simulink model "Simulink_PHEV"  (R2024b)
settings: Solver=VariableStepDiscrete  StartTime=0.0  StopTime=1220  RelTol=1e-3  EnableMultiTasking=on
values from neighbouring files (symbols this model uses):
  eta_EM_map = [0.5831 0.6831 0.781 0.826 0 0 0 0 0 0.6107 0.7107 0.8049 ... (270 elements, 9x30)]    [Initial_Data.mat]
  h = []    [Initial_Data.mat]
  H_u = 42936779.9114    [Initial_Data.mat]
  P_MGB_FTP75 = [0 0 0 0 0 0 0 0 0 0 0 0 ... (1878 elements, 1878x1)]    [Initial_Data.mat]
  PMGB_NEDC = [0 0 0 0 0 0 0 0 0 0 0 0 ... (1221 elements, 1221x1)]    [Initial_Data.mat]
  rho_f = 0.843    [Initial_Data.mat]
  T_CE_max = [118.899401682 131.236739827 143.574077972 164.791588079 186.009098185 184.856709457 183.704320729 184.924497029 186.144673329 186.619186335 187.093699341 186.822549052 ... (31 elements, 1x31)]    [Initial_Data.mat]
  T_EM_max = [60 60 60 44.5714285714 32.5714285714 24 16.2857142857 11.1428571429 7.71428571429]    [Initial_Data.mat]
  V_CE_map = [0.000142 0.000157 0.000171 0.000186 0.000201 0.000215 0.000229 0.000255 0.00028 0.000299 0.000317 0.000346 ... (868 elements, 31x28)]    [Initial_Data.mat]
  w_CE_max = [125.663706144 136.135681656 146.607657168 157.079632679 167.551608191 178.023583703 188.495559215 198.967534727 209.439510239 219.911485751 230.383461263 240.855436775 ... (31 elements, 1x31)]    [Initial_Data.mat]
  w_EM_row = [0 100 200 300 400 500 600 700 800]    [Initial_Data.mat]
undefined symbols (not defined in the file or in its folder): c_BT_E1, c_BT_E2, c_BT_E3, c_BT_E4, c_BT_L1, c_BT_L2, c_BT_L3, c_BT_L4, I_BT_max, Q_BT_0, Q_BT_IC
libraries: qss_tb_library x6, mpclib x1, dspindex x1
settings Model: Creator=d_goerges  LastModifiedBy=mohammed omrez khan
settings SolverCC: AlgebraicLoopSolver=TrustRegion
settings DataIOCC: LimitDataPoints=on  SaveFormat=Array  SignalLoggingSaveFormat=ModelDataLogs  ReturnWorkspaceOutputs=off
settings OptimizationCC: ExpressionDepthLimit=2147483647  LifeSpan=inf
settings DebuggingCC: MergeDetectMultiDrivingBlocksExec=none  SolverPrmCheckMsg=warning  FcnCallInpInsideContextMsg=warning  UnconnectedInputMsg=warning  UnconnectedOutputMsg=warning  UnconnectedLineMsg=warning  StateNameClashWarn=warning  SFUnexpectedBacktrackingDiag=warning  SFNoUnconditionalDefaultTransitionDiag=warning  SFExecutionAtInitializationDiag=none  UnderSpecifiedDimensionMsg=warning  ArithmeticOperatorsInVariantConditions=warning
settings HardwareCC: ProdBitPerPointer=32  ProdBitPerSizeT=32  ProdBitPerPtrDiffT=32  ProdLargestAtomicFloat=None  ProdIntDivRoundTo=Undefined  ProdEndianess=Unspecified  ProdWordSize=32  ProdHWDeviceType=32-bit Generic
settings ModelReferenceCC: PropagateSignalLabelsOutOfModel=off
settings SFSimCC: SimUseLocalCustomCode=off  CustomCodeUndefinedFunction=UseInterfaceOnly
settings RTWCC: RTWUseLocalCustomCode=off  GPUComputeCapability=3.5
settings CodeAppCC: StateflowObjectComments=on
settings GRTTargetCC: TargetLangStandard=C89/C90 (ANSI)  CombineOutputUpdateFcns=off  GRTInterface=on
settings ConfigComp: CovMetricSettings=dw  CovSaveCumulativeToWorkspaceVar=on  CovSaveSingleToWorkspaceVar=on  CovExternalEMLEnable=off

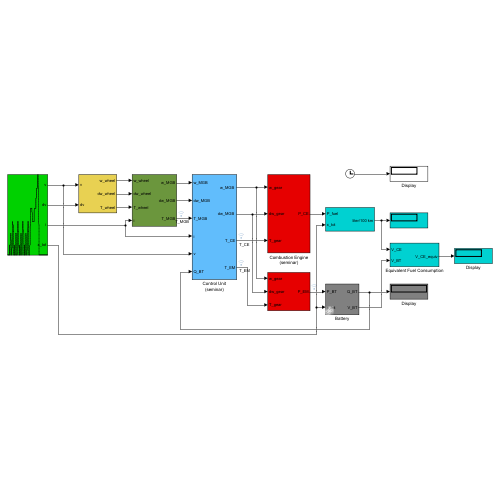
[thumbnail: Simulink's stored preview of the top-level diagram]
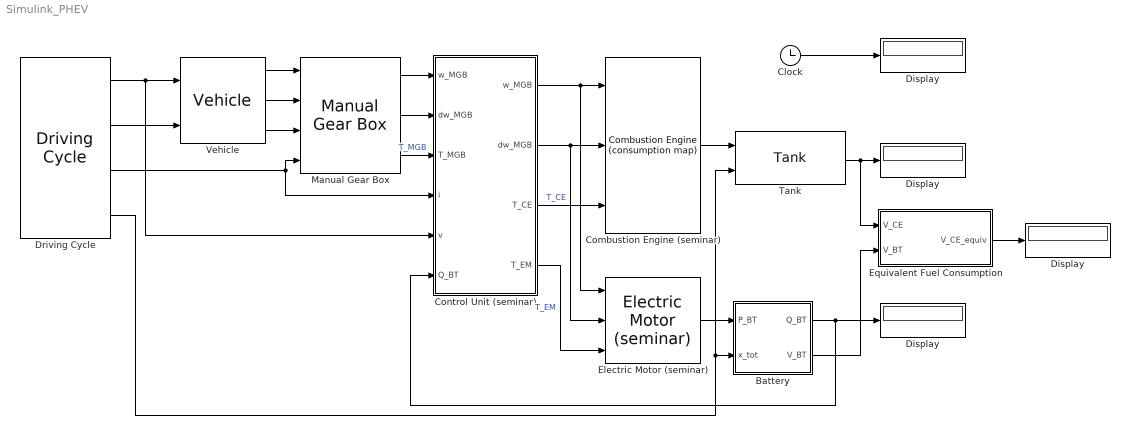
== system Simulink_PHEV ==
  "   Display   " : Display
  "  Display  " : Display
  " Display " : Display
  Battery : Subsystem  Tag=battery  AncestorBlock=qss_tb_library/Energy Buffer/Battery  mask(Battery){I_0=10, Q_BT_IC_rel=50, t_ch=2}
      mask prompts: I_0 "Energy capacity of battery [Ah]"; Q_BT_IC_rel "Initial charge of battery [%]"; t_ch "Current limit: minimum time to charge/discharge the battery [min]"
      mask help:
      | This block simulates a battery.
      | The resistance depends on the charge state and the charge/discharge current of the battery. The battery has an open circuit voltage of 130 V (fully charged).
      |
      | Input:
      | =====
      | 	x_tot	Total distance [m]
      | 	P_BT	Power from/to the battery [W]
      | 		P_BT < 0: battery charging
      | 		P_BT > 0: battery discharging
      |
      | Output:
      | ======
      | 	Q_BT	Current charge of the battery [C]
      | 	V_BT	Energy consumption [kWh/100 km]
      mask init:
      | init_BT;
  Clock : Clock
  Combustion Engine (seminar) : qss_tb_library/Energy Converter/Combustion Engine (consumption map)  Tag=combustion engine  theta_CE=0.2  w_CE_idle=105  P_CE_idle=8000  P_aux=0  ENABLE_FUEL_CUTOFF=on  T_CE_cutoff=5  P_CE_cutoff=0
  Control Unit (seminar) : Subsystem  Tag=control unit  mask(Control Unit){}
      mask help:
      | This block gives the user the opportunity to design his/her own control unit.
      |
      | The user can define the inputs and outputs  by himself/herself.
      mask init:
      | %init_control_unit;
  Display : Display
  Driving Cycle : qss_tb_library/Driving Cycle/Driving Cycle  Tag=cycle  cyclenr=Europe: NEDC  stepsize=1  autostop=on
  Electric Motor (seminar) : qss_tb_library/Energy Converter/Electric Motor (seminar)  theta_EM=0.1  P_aux=0
  Equivalent Fuel Consumption : Subsystem  mask(Equivalent Fuel Consumption){eta_BT=0.9, eta_EM=0.8, eta_CE=0.25}
      mask prompts: eta_BT "Battery efficiency [-]"; eta_EM "Motor efficiency [-]"; eta_CE "Engine efficiency [-]"
      mask help:
      | This block computes the equivalent fuel consumption.
      |
      | Input:
      | =====
      | 	V_CE    Fuel consumption [l/100 km]
      | 	V_BT    Energy consumption [kWh/100 km]
      |
      | Output:
      | ======
      | 	V_CE_equiv	Equivalent fuel consumption [l/100 km]
      mask init:
      | init_equivalent_fuel_consumption;
  Manual Gear Box : qss_tb_library/Gear System/Manual Gear Box  Tag=transmission  i_1=3.27  i_2=1.92  i_3=1.26  i_4=0.88  i_5=0.7  i_diff=3.29  e_GT=0.98  P_GT0=100  w_wheel_min=1
  Tank : qss_tb_library/Energy Source/Tank  Tag=tank  fuel=Diesel  flag_cold_start=on
  Vehicle : qss_tb_library/Vehicle/Vehicle  Tag=vehicle  m_f=1115  mt2m_f=5  A_f=2.3  d_wheel=0.576  cw=0.31  mu=0.013
  wires:
  Tank/1 -> Display/1, Equivalent Fuel Consumption/1(V_CE)
  Driving Cycle/2 -> Vehicle/2
  Driving Cycle/1 -> Vehicle/1, Control Unit (seminar)/5(v)
  Vehicle/1 -> Manual Gear Box/1
  Vehicle/2 -> Manual Gear Box/2
  Vehicle/3 -> Manual Gear Box/3
  Manual Gear Box/1 -> Control Unit (seminar)/1(w_MGB)
  Manual Gear Box/2 -> Control Unit (seminar)/2(dw_MGB)
  Manual Gear Box/3 -> Control Unit (seminar)/3(T_MGB)  "T_MGB"
  Control Unit (seminar)/1(" w_MGB ") -> Combustion Engine (seminar)/1, Electric Motor (seminar)/1
  Control Unit (seminar)/2(" dw_MGB ") -> Combustion Engine (seminar)/2, Electric Motor (seminar)/2
  Control Unit (seminar)/3(T_CE) -> Combustion Engine (seminar)/3  "T_CE"
  Control Unit (seminar)/4(T_EM) -> Electric Motor (seminar)/3  "T_EM"
  Combustion Engine (seminar)/1 -> Tank/1
  Electric Motor (seminar)/1 -> Battery/1(P_BT)
  Driving Cycle/4 -> Battery/2(x_tot), Tank/2
  Battery/1(Q_BT) -> "  Display  "/1, Control Unit (seminar)/6(Q_BT)
  Driving Cycle/3 -> Manual Gear Box/4, Control Unit (seminar)/4(i)
  Battery/2(V_BT) -> Equivalent Fuel Consumption/2(V_BT)
  Clock/1 -> " Display "/1
  Equivalent Fuel Consumption/1(V_CE_equiv) -> "   Display   "/1

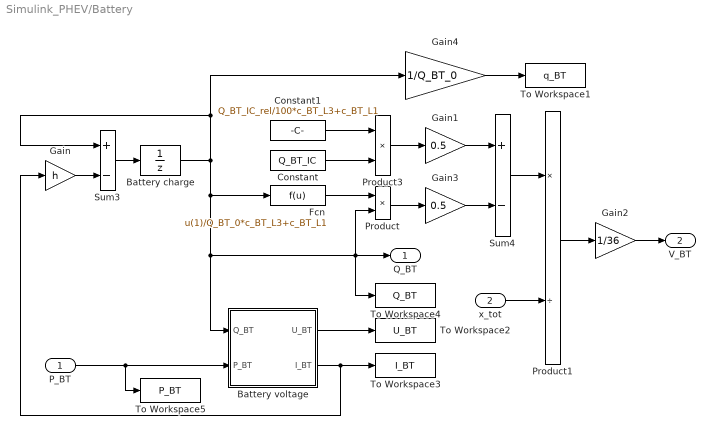
== system Simulink_PHEV/Battery ==
  P_BT : Inport
  x_tot : Inport  Port=2
  Battery charge : UnitDelay  InitialCondition=Q_BT_IC  SampleTime=h  HasFrameUpgradeWarning=on
  Battery voltage : Subsystem
  Constant : Constant  Value=Q_BT_IC
  Constant1 : Constant  Value=Q_BT_IC_rel/100*c_BT_L3+c_BT_L1
  Fcn : Fcn  Expr=u(1)/Q_BT_0*c_BT_L3+c_BT_L1
  Gain : Gain  Gain=h  SaturateOnIntegerOverflow=on  OutDataTypeStr=Inherit: Same as input  ParamDataTypeStr=Inherit: Same as input
  Gain1 : Gain  Gain=0.5  SaturateOnIntegerOverflow=on  OutDataTypeStr=Inherit: Same as input  ParamDataTypeStr=Inherit: Same as input
  Gain2 : Gain  Gain=1/36  SaturateOnIntegerOverflow=on  OutDataTypeStr=Inherit: Same as input  ParamDataTypeStr=Inherit: Same as input
  Gain3 : Gain  Gain=0.5  SaturateOnIntegerOverflow=on  OutDataTypeStr=Inherit: Same as input  ParamDataTypeStr=Inherit: Same as input
  Gain4 : Gain  Gain=1/Q_BT_0  SaturateOnIntegerOverflow=on  OutDataTypeStr=Inherit: Same as input  ParamDataTypeStr=Inherit: Same as input
  Product : Product  RndMeth=Zero
  Product1 : Product  Inputs=*/  InputSameDT=on  RndMeth=Zero  SaturateOnIntegerOverflow=on  OutDataTypeStr=Inherit: Same as first input
  Product3 : Product  RndMeth=Zero
  Sum3 : Sum  Inputs=+-  InputSameDT=on  SaturateOnIntegerOverflow=on  OutDataTypeStr=Inherit: Same as first input
  Sum4 : Sum  Inputs=+-  InputSameDT=on  SaturateOnIntegerOverflow=on  OutDataTypeStr=Inherit: Same as first input
  To Workspace1 : ToWorkspace  VariableName=q_BT  SampleTime=-1
  To Workspace2 : ToWorkspace  VariableName=U_BT  SampleTime=-1
  To Workspace3 : ToWorkspace  VariableName=I_BT  SampleTime=-1
  To Workspace4 : ToWorkspace  VariableName=Q_BT  SampleTime=-1
  To Workspace5 : ToWorkspace  VariableName=P_BT  SampleTime=-1
  Q_BT : Outport  InitialOutput=0
  V_BT : Outport  Port=2  InitialOutput=0
  wires:
  Fcn/1 -> Product/1
  Constant1/1 -> Product3/1
  Constant/1 -> Product3/2
  Gain2/1 -> V_BT/1
  Sum4/1 -> Product1/1
  Gain3/1 -> Sum4/2
  Gain1/1 -> Sum4/1
  Product/1 -> Gain3/1
  Product3/1 -> Gain1/1
  P_BT/1 -> To Workspace5/1, Battery voltage/2(P_BT)
  Gain4/1 -> To Workspace1/1
  Product1/1 -> Gain2/1
  x_tot/1 -> Product1/2
  Battery voltage/1(U_BT) -> To Workspace2/1
  Battery charge/1 -> Fcn/1, To Workspace4/1, Q_BT/1, Product/2, Battery voltage/1(Q_BT), Gain4/1, Sum3/1
  Gain/1 -> Sum3/2
  Sum3/1 -> Battery charge/1
  Battery voltage/2(I_BT) -> To Workspace3/1, Gain/1

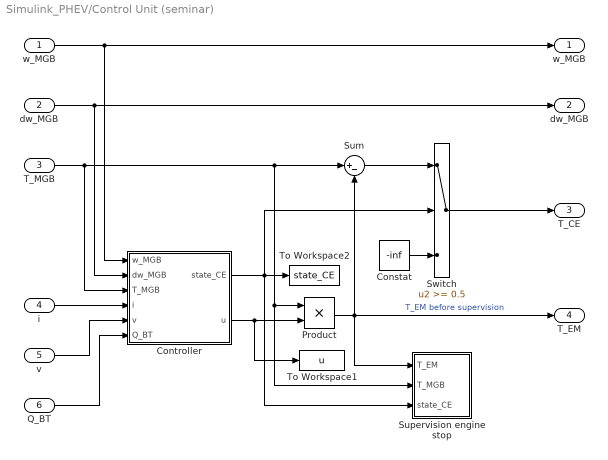
== system Simulink_PHEV/Control Unit (seminar) ==
  w_MGB : Inport
  dw_MGB : Inport  Port=2
  T_MGB : Inport  Port=3
  i : Inport  Port=4
  v : Inport  Port=5
  Q_BT : Inport  Port=6
  Constat : Constant  Value=-inf
  Controller : Subsystem  TreatAsAtomicUnit=on
  Product : Product  RndMeth=Zero
  Sum : Sum  Inputs=|+-
  Supervision engine stop : Subsystem
  Switch : Switch  Threshold=0.5  SaturateOnIntegerOverflow=off  InputSameDT=off
  To Workspace1 : ToWorkspace  VariableName=u  SampleTime=-1
  To Workspace2 : ToWorkspace  VariableName=state_CE  SampleTime=-1
  " w_MGB " : Outport  InitialOutput=0
  " dw_MGB " : Outport  Port=2  InitialOutput=0
  T_CE : Outport  Port=3  InitialOutput=0
  T_EM : Outport  Port=4  InitialOutput=0
  wires:
  dw_MGB/1 -> Controller/2(dw_MGB), " dw_MGB "/1
  w_MGB/1 -> Controller/1(w_MGB), " w_MGB "/1
  T_MGB/1 -> Controller/3(T_MGB), Sum/1, Product/1, Supervision engine stop/2(T_MGB)
  Product/1 -> Sum/2, T_EM/1, Supervision engine stop/1(T_EM)  "T_EM before supervision"
  i/1 -> Controller/4(i)
  Controller/1(state_CE) -> Switch/2, To Workspace2/1, Supervision engine stop/3(state_CE)
  Sum/1 -> Switch/1
  Switch/1 -> T_CE/1
  Constat/1 -> Switch/3
  v/1 -> Controller/5(v)
  Q_BT/1 -> Controller/6(Q_BT)
  Controller/2(u) -> To Workspace1/1, Product/2

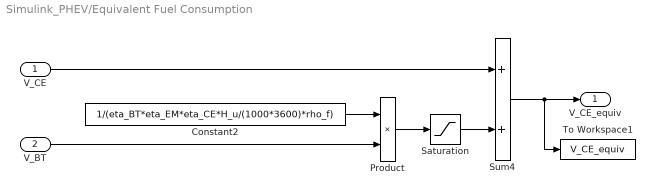
== system Simulink_PHEV/Equivalent Fuel Consumption ==
  V_CE : Inport
  V_BT : Inport  Port=2
  Constant2 : Constant  Value=1/(eta_BT*eta_EM*eta_CE*H_u/(1000*3600)*rho_f)
  Product : Product  RndMeth=Zero
  Saturation : Saturate  UpperLimit=inf  LowerLimit=0
  Sum4 : Sum  InputSameDT=on  SaturateOnIntegerOverflow=on  OutDataTypeStr=Inherit: Same as first input
  To Workspace1 : ToWorkspace  VariableName=V_CE_equiv  SampleTime=-1
  V_CE_equiv : Outport
  wires:
  Product/1 -> Saturation/1
  V_BT/1 -> Product/2
  Constant2/1 -> Product/1
  Sum4/1 -> To Workspace1/1, V_CE_equiv/1
  V_CE/1 -> Sum4/1
  Saturation/1 -> Sum4/2

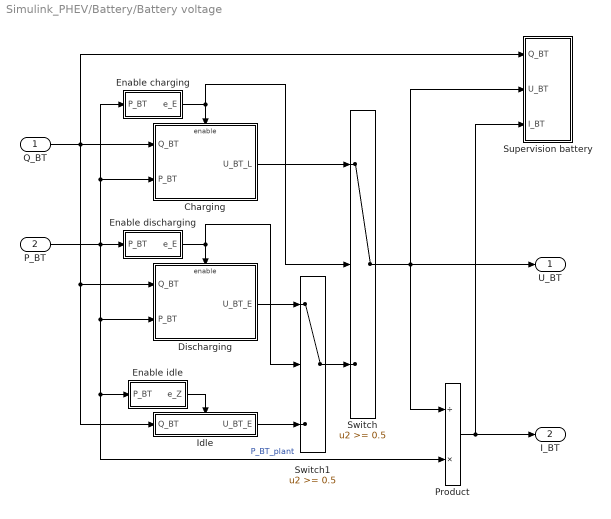
== system Simulink_PHEV/Battery/Battery voltage ==
  Q_BT : Inport
  P_BT : Inport  Port=2
  Charging : Subsystem
  Discharging : Subsystem
  Enable charging : Subsystem
  Enable discharging : Subsystem
  Enable idle : Subsystem
  Idle : Subsystem
  Product : Product  Inputs=/*  InputSameDT=on  RndMeth=Zero  SaturateOnIntegerOverflow=on  OutDataTypeStr=Inherit: Same as first input
  Supervision battery : Subsystem
  Switch : Switch  Threshold=0.5
  Switch1 : Switch  Threshold=0.5
  U_BT : Outport  InitialOutput=0
  I_BT : Outport  Port=2  InitialOutput=0
  wires:
  Switch/1 -> U_BT/1, Supervision battery/2(U_BT), Product/1
  Enable charging/1(e_E) -> Switch/2, Charging/Enable
  Q_BT/1 -> Idle/1(Q_BT), Discharging/1(Q_BT), Charging/1(Q_BT), Supervision battery/1(Q_BT)
  Product/1 -> I_BT/1, Supervision battery/3(I_BT)
  Enable discharging/1(e_E) -> Switch1/2, Discharging/Enable
  P_BT/1 -> Enable discharging/1(P_BT), Discharging/2(P_BT), Product/2, Enable idle/1(P_BT), Enable charging/1(P_BT), Charging/2(P_BT)  "P_BT_plant"
  Discharging/1(U_BT_E) -> Switch1/1
  Idle/1(U_BT_E) -> Switch1/3
  Switch1/1 -> Switch/3
  Charging/1(U_BT_L) -> Switch/1
  Enable idle/1(e_Z) -> Idle/Enable

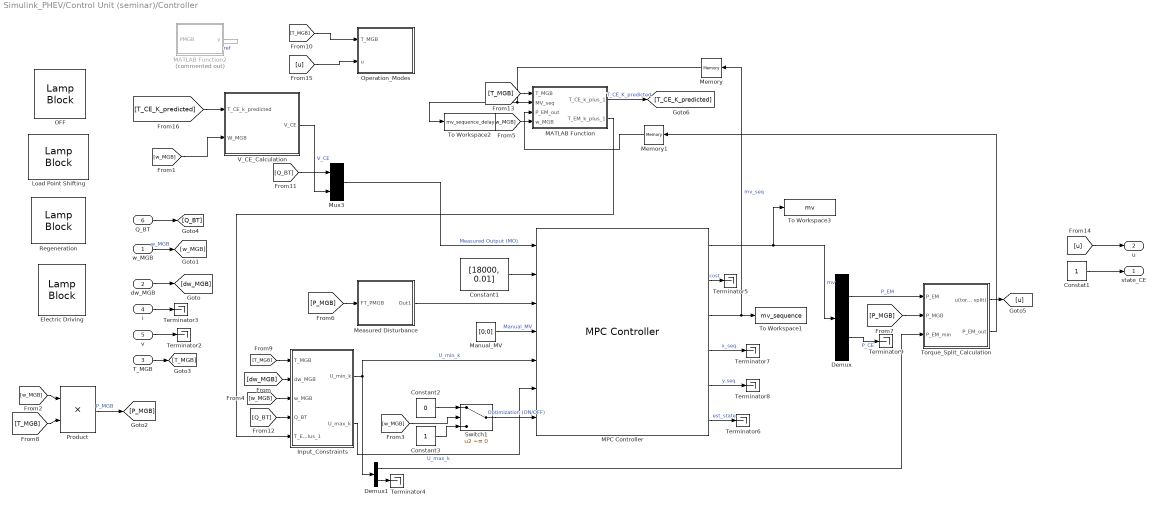
== system Simulink_PHEV/Control Unit (seminar)/Controller ==
  w_MGB : Inport
  dw_MGB : Inport  Port=2
  T_MGB : Inport  Port=3
  i : Inport  Port=4
  v : Inport  Port=5
  Q_BT : Inport  Port=6
  Constant1 : Constant  Value=[18000, 0.01]  VectorParams1D=off
  Constant2 : Constant  Value=0
  Constant3 : Constant
  Constat1 : Constant
  Demux : Demux  Outputs=2
  Demux1 : Demux  Outputs=2
  Electric Driving : LampBlock  LabelPosition=Hide
  Input_Constraints : Subsystem
  "Load Point Shifting " : LampBlock  LabelPosition=Hide
  MATLAB Function : MATLAB Function  TreatAsAtomicUnit=on
  MATLAB Function2 : MATLAB Function  Commented=on  TreatAsAtomicUnit=on
  MPC Controller : mpclib/MPC Controller  SCDEnableBlockLinearizationSpecification=on  mpcobj=mpc_object  is_multiple=0  enable_value=0  return_u0=off  updateMPCinCallerWorkspace=on  md_inport=on  mv_inport=on  uref_inport=off  return_cost=on  return_mvseq=on  return_qpstatus=off  return_xseq=on  return_state=on  return_ovseq=on  state_inport=off  umin_inport=on  umax_inport=on  ymin_inport=off  ymax_inport=off  cc_inport=off  ywt_inport=off  uwt_inport=off  duwt_inport=off  rhoeps_inport=off  pm_inport=off  MaximumP=10  HorizonChoice=FixedHorizon  n_ts=1  n_p=11  n_mv=2  n_md=1  n_ud=0  n_mo=2  n_uo=0  BlockDataType=double  SampleTimeInherited=off  switch_inport=on
  Manual_MV : Constant  Value=[0;0]  VectorParams1D=off
  Measured Disturbance : Subsystem
  Memory : Memory
  Memory1 : Memory
  Mux3 : Mux  Inputs=2
  OFF : LampBlock  LabelPosition=Hide
  Operation_Modes : Stateflow chart  TreatAsAtomicUnit=on
  Product : Product  OutDataTypeStr=double
  Regeneration : LampBlock  LabelPosition=Hide
  Switch1 : Switch  Criteria=u2 ~= 0  SaturateOnIntegerOverflow=off  InputSameDT=off
  Terminator{2..9} (8 alike) : Terminator
  To Workspace1 : ToWorkspace  VariableName=mv_sequence  SaveFormat=Timeseries  SampleTime=-1
  To Workspace2 : ToWorkspace  VariableName=mv_sequence_delay  SaveFormat=Timeseries  SampleTime=-1
  To Workspace3 : ToWorkspace  VariableName=mv  SaveFormat=Timeseries  SampleTime=-1
  Torque_Split_Calculation : Subsystem
  V_CE_Calculation : Subsystem
  state_CE : Outport  InitialOutput=0
  u : Outport  Port=2  InitialOutput=0
  wires:
  dw_MGB/1 -> [dw_MGB]
  i/1 -> Terminator3/1
  Product/1 -> [P_MGB]  "P_MGB"
  V_CE_Calculation/1(V_CE) -> Mux3/2  "V_CE"
  Input_Constraints/1(U_min_k) -> MPC Controller/5, Demux1/1  "U_min_k"
  Input_Constraints/2(U_max_k) -> MPC Controller/6  "U_max_k"
  Demux/1 -> Torque_Split_Calculation/1(P_EM)  "P_EM"
  Mux3/1 -> MPC Controller/1  "Measured Output (MO)"
  Constant1/1 -> MPC Controller/2
  v/1 -> Terminator2/1
  MPC Controller/1 -> To Workspace3/1, Demux/1  "mv"
  Manual_MV/1 -> MPC Controller/4  "Manual_MV"
  Demux/2 -> Terminator9/1  "P_CE"
  Switch1/1 -> MPC Controller/7  "Optimization (ON/OFF)"
  Constant2/1 -> Switch1/1
  Constant3/1 -> Switch1/3
  Demux1/1 -> Torque_Split_Calculation/3(P_EM_min)
  Demux1/2 -> Terminator4/1
  MPC Controller/5 -> Terminator8/1  "y.seq"
  MPC Controller/3 -> Memory/1, To Workspace1/1  "mv_seq"
  MPC Controller/6 -> Terminator6/1  "est_state"
  MPC Controller/4 -> Terminator7/1  "x_seq"
  MPC Controller/2 -> Terminator5/1  "cost"
  Memory/1 -> To Workspace2/1, MATLAB Function/2(MV_seq)
  Constat1/1 -> state_CE/1
  MATLAB Function/2(T_EM_k_plus_1) -> Input_Constraints/5(T_EM_k_plus_1)
  MATLAB Function2/1(y) -> ?  "ref"
  [dw_MGB] -> Input_Constraints/2(dw_MGB)
  w_MGB/1 -> [w_MGB]  "w_MGB"
  [w_MGB] -> V_CE_Calculation/2(W_MGB)
  [w_MGB] -> Product/1
  [w_MGB] -> Switch1/2
  [w_MGB] -> Input_Constraints/3(w_MGB)
  [w_MGB] -> MATLAB Function/4(w_MGB)
  [P_MGB] -> Measured Disturbance/1(FT_PMGB)
  [P_MGB] -> Torque_Split_Calculation/2(P_MGB)
  T_MGB/1 -> [T_MGB]
  [T_MGB] -> Product/2
  [T_MGB] -> Input_Constraints/1(T_MGB)
  [T_MGB] -> Operation_Modes/1(T_MGB)
  Measured Disturbance/1(Out1) -> MPC Controller/3
  Q_BT/1 -> [Q_BT]
  [Q_BT] -> Mux3/1
  [Q_BT] -> Input_Constraints/4(Q_BT)
  Memory1/1 -> MATLAB Function/3(P_EM_out)
  [T_MGB] -> MATLAB Function/1(T_MGB)
  Torque_Split_Calculation/2(P_EM_out) -> Memory1/1
  Torque_Split_Calculation/1(u(torque split)) -> [u]
  [u] -> u/1
  [u] -> Operation_Modes/2(u)
  MATLAB Function/1(T_CE_k_plus_1) -> [T_CE_K_predicted]  "T_CE_K_predicted"
  [T_CE_K_predicted] -> V_CE_Calculation/1(T_CE_k_predicted)

== system Simulink_PHEV/Control Unit (seminar)/Supervision engine stop ==
  T_EM : Inport
  T_MGB : Inport  Port=2
  state_CE : Inport  Port=3
  Interpreted MATLAB Function : MATLABFcn  MATLABFcn=supervision_engine_stop
  Mux : Mux  Inputs=3
  Stop Simulation : Stop
  wires:
  T_MGB/1 -> Mux/2
  T_EM/1 -> Mux/1
  state_CE/1 -> Mux/3
  Mux/1 -> Interpreted MATLAB Function/1
  Interpreted MATLAB Function/1 -> Stop Simulation/1  "Overload_supervision"

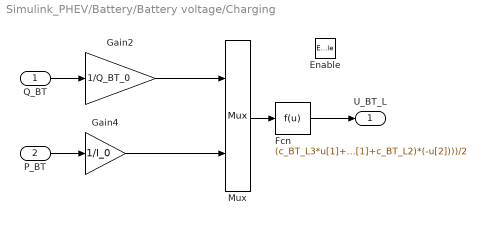
== system Simulink_PHEV/Battery/Battery voltage/Charging ==
  Q_BT : Inport
  P_BT : Inport  Port=2
  Enable : EnablePort
  Fcn : Fcn  Expr=(c_BT_L3*u[1]+c_BT_L1+sqrt((c_BT_L3*u[1]+c_BT_L1)^2+4*(c_BT_L4*u[1]+c_BT_L2)*(-u[2])))/2
  Gain2 : Gain  Gain=1/Q_BT_0  SaturateOnIntegerOverflow=on  OutDataTypeStr=Inherit: Same as input  ParamDataTypeStr=Inherit: Same as input
  Gain4 : Gain  Gain=1/I_0  SaturateOnIntegerOverflow=on  OutDataTypeStr=Inherit: Same as input  ParamDataTypeStr=Inherit: Same as input
  Mux : Mux  Inputs=2
  U_BT_L : Outport  InitialOutput=0
  wires:
  Fcn/1 -> U_BT_L/1
  Mux/1 -> Fcn/1
  P_BT/1 -> Gain4/1
  Q_BT/1 -> Gain2/1
  Gain2/1 -> Mux/1
  Gain4/1 -> Mux/2

== system Simulink_PHEV/Battery/Battery voltage/Discharging ==
  note: P/I_0
  note: q
  Q_BT : Inport
  P_BT : Inport  Port=2
  Enable : EnablePort
  Fcn : Fcn  Expr=(c_BT_E3*u[1]+c_BT_E1+sqrt((c_BT_E3*u[1]+c_BT_E1)^2+4*(c_BT_E4*u[1]+c_BT_E2)*(-u[2])))/2
  Gain4 : Gain  Gain=1/Q_BT_0  SaturateOnIntegerOverflow=on  OutDataTypeStr=Inherit: Same as input  ParamDataTypeStr=Inherit: Same as input
  Gain5 : Gain  Gain=1/I_0  SaturateOnIntegerOverflow=on  OutDataTypeStr=Inherit: Same as input  ParamDataTypeStr=Inherit: Same as input
  Mux : Mux  Inputs=2
  U_BT_E : Outport  InitialOutput=0
  wires:
  Mux/1 -> Fcn/1
  Gain5/1 -> Mux/2
  Gain4/1 -> Mux/1
  P_BT/1 -> Gain5/1
  Q_BT/1 -> Gain4/1
  Fcn/1 -> U_BT_E/1

== system Simulink_PHEV/Battery/Battery voltage/Enable charging ==
  P_BT : Inport
  Gain : Gain  Gain=-1  SaturateOnIntegerOverflow=on  OutDataTypeStr=Inherit: Same as input  ParamDataTypeStr=Inherit: Same as input
  Saturation : Saturate  UpperLimit=0  LowerLimit=-inf
  Sign : Signum
  e_E : Outport  InitialOutput=0
  wires:
  Gain/1 -> Sign/1
  Saturation/1 -> Gain/1
  Sign/1 -> e_E/1
  P_BT/1 -> Saturation/1

== system Simulink_PHEV/Battery/Battery voltage/Enable discharging ==
  P_BT : Inport
  Saturation : Saturate  UpperLimit=inf  LowerLimit=0
  Sign : Signum
  e_E : Outport  InitialOutput=0
  wires:
  Saturation/1 -> Sign/1
  Sign/1 -> e_E/1
  P_BT/1 -> Saturation/1

== system Simulink_PHEV/Battery/Battery voltage/Enable idle ==
  P_BT : Inport
  Abs : Abs
  Constant : Constant
  Sign : Signum
  Sum4 : Sum  Inputs=-+  InputSameDT=on  SaturateOnIntegerOverflow=on  OutDataTypeStr=Inherit: Same as first input
  e_Z : Outport  InitialOutput=0
  wires:
  Constant/1 -> Sum4/2
  Sum4/1 -> e_Z/1
  Abs/1 -> Sum4/1
  Sign/1 -> Abs/1
  P_BT/1 -> Sign/1

== system Simulink_PHEV/Battery/Battery voltage/Idle ==
  Q_BT : Inport
  Enable : EnablePort  StatesWhenEnabling=reset
  Constant : Constant  Value=c_BT_L1
  Gain4 : Gain  Gain=c_BT_L3/Q_BT_0  SaturateOnIntegerOverflow=on  OutDataTypeStr=Inherit: Same as input  ParamDataTypeStr=Inherit: Same as input
  Sum8 : Sum  InputSameDT=on  SaturateOnIntegerOverflow=on  OutDataTypeStr=Inherit: Same as first input
  U_BT_E : Outport  InitialOutput=0
  wires:
  Sum8/1 -> U_BT_E/1
  Constant/1 -> Sum8/2
  Gain4/1 -> Sum8/1
  Q_BT/1 -> Gain4/1

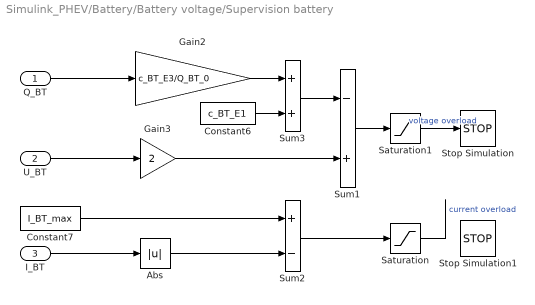
== system Simulink_PHEV/Battery/Battery voltage/Supervision battery ==
  Q_BT : Inport
  U_BT : Inport  Port=2
  I_BT : Inport  Port=3
  Abs : Abs
  Constant6 : Constant  Value=c_BT_E1
  Constant7 : Constant  Value=I_BT_max
  Gain2 : Gain  Gain=c_BT_E3/Q_BT_0  SaturateOnIntegerOverflow=on  OutDataTypeStr=Inherit: Same as input  ParamDataTypeStr=Inherit: Same as input
  Gain3 : Gain  Gain=2  SaturateOnIntegerOverflow=on  OutDataTypeStr=Inherit: Same as input  ParamDataTypeStr=Inherit: Same as input
  Saturation : Saturate  UpperLimit=0  LowerLimit=-inf
  Saturation1 : Saturate  UpperLimit=0  LowerLimit=-inf
  Stop Simulation : Stop
  Stop Simulation1 : Stop
  Sum1 : Sum  Inputs=-+  InputSameDT=on  SaturateOnIntegerOverflow=on  OutDataTypeStr=Inherit: Same as first input
  Sum2 : Sum  Inputs=+-  InputSameDT=on  SaturateOnIntegerOverflow=on  OutDataTypeStr=Inherit: Same as first input
  Sum3 : Sum  InputSameDT=on  SaturateOnIntegerOverflow=on  OutDataTypeStr=Inherit: Same as first input
  wires:
  Q_BT/1 -> Gain2/1
  Abs/1 -> Sum2/2
  I_BT/1 -> Abs/1
  Sum2/1 -> Saturation/1
  Constant7/1 -> Sum2/1
  Gain2/1 -> Sum3/1
  Constant6/1 -> Sum3/2
  Sum1/1 -> Saturation1/1
  Saturation1/1 -> Stop Simulation/1  "voltage overload"
  Saturation/1 -> ?  "current overload"
  Gain3/1 -> Sum1/2
  U_BT/1 -> Gain3/1
  Sum3/1 -> Sum1/1

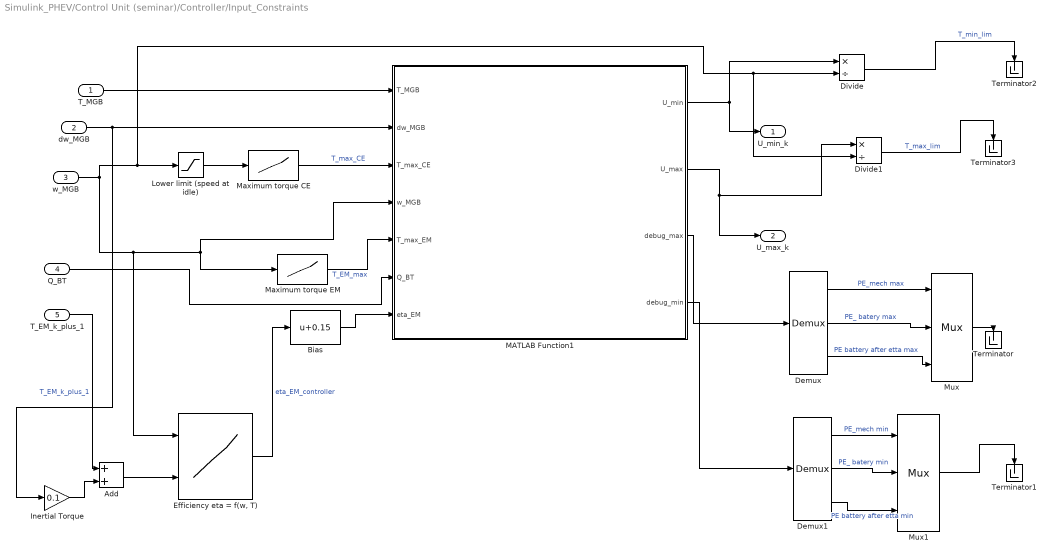
== system Simulink_PHEV/Control Unit (seminar)/Controller/Input_Constraints ==
  T_MGB : Inport
  dw_MGB : Inport  Port=2
  w_MGB : Inport  Port=3
  Q_BT : Inport  Port=4
  T_EM_k_plus_1 : Inport  Port=5
  Add : Sum
  Bias : Bias  Bias=0.15  SaturateOnIntegerOverflow=off
  Demux : Demux  Outputs=3
  Demux1 : Demux  Outputs=3
  Divide : Product  Inputs=*/
  Divide1 : Product  Inputs=*/
  "Efficiency eta = f(w, T)" : Lookup2D  RowIndex=w_EM_row  ColumnIndex=T_EM_col  Table=eta_EM_map  InputSameDT=off
  Inertial Torque : Gain  Gain=0.1
  Lower limit (speed at idle) : Saturate  UpperLimit=inf  LowerLimit=105
  MATLAB Function1 : MATLAB Function  TreatAsAtomicUnit=on
  Maximum torque CE : Lookup  InputValues=w_CE_max  Table=T_CE_max
  Maximum torque EM : Lookup  InputValues=w_EM_row  Table=T_EM_max
  Mux : Mux  Inputs=3
  Mux1 : Mux  Inputs=3
  Terminator{,1..3} (4 alike) : Terminator
  U_min_k : Outport
  U_max_k : Outport  Port=2
  wires:
  w_MGB/1 -> "Efficiency eta = f(w, T)"/1, MATLAB Function1/4(w_MGB), Maximum torque EM/1, Divide1/2, Divide/2, Lower limit (speed at idle)/1
  Maximum torque CE/1 -> MATLAB Function1/3(T_max_CE)  "T_max_CE"
  Maximum torque EM/1 -> MATLAB Function1/5(T_max_EM)  "T_EM_max"
  Lower limit (speed at idle)/1 -> Maximum torque CE/1
  dw_MGB/1 -> Inertial Torque/1, MATLAB Function1/2(dw_MGB)
  T_MGB/1 -> MATLAB Function1/1(T_MGB)
  MATLAB Function1/1(U_min) -> U_min_k/1, Divide/1
  MATLAB Function1/2(U_max) -> Divide1/1, U_max_k/1
  Q_BT/1 -> MATLAB Function1/6(Q_BT)
  MATLAB Function1/3(debug_max) -> Demux/1
  Mux/1 -> Terminator/1
  Demux/1 -> Mux/1  "PE_mech max"
  Demux/2 -> Mux/2  "PE_ batery max"
  Demux/3 -> Mux/3  "PE battery after etta max"
  Demux1/3 -> Mux1/3  "PE battery after etta min"
  MATLAB Function1/4(debug_min) -> Demux1/1
  Demux1/1 -> Mux1/1  "PE_mech min"
  Demux1/2 -> Mux1/2  "PE_ batery min"
  Mux1/1 -> Terminator1/1
  "Efficiency eta = f(w, T)"/1 -> Bias/1  "eta_EM_controller"
  T_EM_k_plus_1/1 -> Add/1  "T_EM_k_plus_1"
  Bias/1 -> MATLAB Function1/7(eta_EM)
  Inertial Torque/1 -> Add/2
  Add/1 -> "Efficiency eta = f(w, T)"/2
  Divide/1 -> Terminator2/1  "T_min_lim"
  Divide1/1 -> Terminator3/1  "T_max_lim"

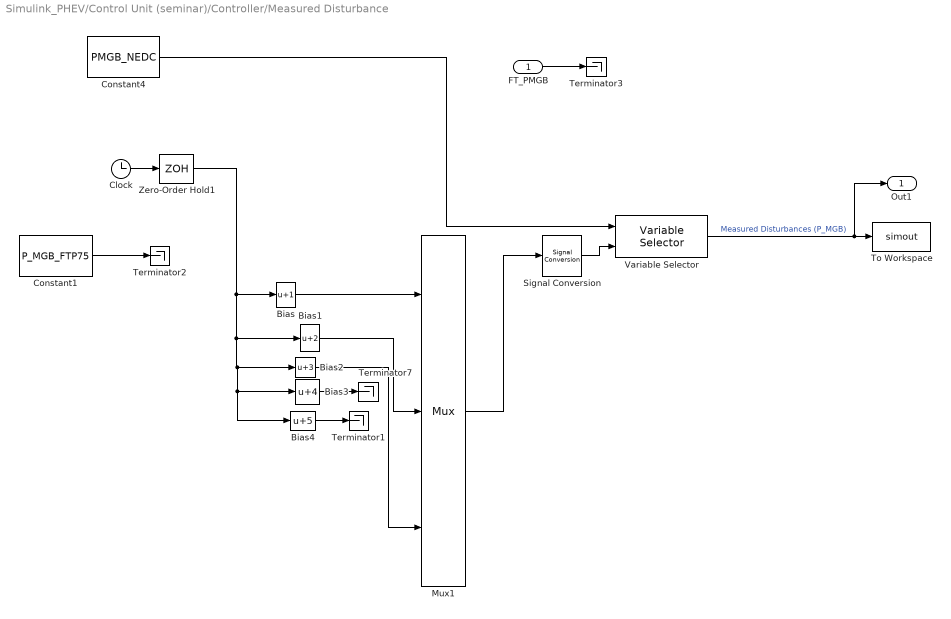
== system Simulink_PHEV/Control Unit (seminar)/Controller/Measured Disturbance ==
  FT_PMGB : Inport
  Bias : Bias  Bias=1  SaturateOnIntegerOverflow=off
  Bias1 : Bias  Bias=2  SaturateOnIntegerOverflow=off
  Bias2 : Bias  Bias=3  SaturateOnIntegerOverflow=off
  Bias3 : Bias  Bias=4  SaturateOnIntegerOverflow=off
  Bias4 : Bias  Bias=5  SaturateOnIntegerOverflow=off
  Clock : Clock
  Constant1 : Constant  Value=P_MGB_FTP75
  Constant4 : Constant  Value=PMGB_NEDC
  Mux1 : Mux  Inputs=3
  Signal Conversion : SignalConversion  OverrideOpt=off
  Terminator{1..3,7} (4 alike) : Terminator
  To Workspace : ToWorkspace  VariableName=simout  SaveFormat=Timeseries  SampleTime=-1
  Variable Selector : dspindex/Variable Selector  NumInputs=1  rowsOrCols=Rows  IdxMode=Variable  Elements=[1 3]  ZerOneIdxMode=One-based  errmode=Clip Index  FillMode=on  FillValues=0
  Zero-Order Hold1 : ZeroOrderHold  SampleTime=-1
  Out1 : Outport
  wires:
  Bias4/1 -> Terminator1/1
  Bias3/1 -> Terminator7/1
  Bias/1 -> Mux1/1
  Mux1/1 -> Signal Conversion/1
  Clock/1 -> Zero-Order Hold1/1
  Bias2/1 -> Mux1/3
  Variable Selector/1 -> Out1/1, To Workspace/1  "Measured Disturbances (P_MGB)"
  Bias1/1 -> Mux1/2
  Signal Conversion/1 -> Variable Selector/2
  Zero-Order Hold1/1 -> Bias2/1, Bias4/1, Bias3/1, Bias1/1, Bias/1
  Constant1/1 -> Terminator2/1
  Constant4/1 -> Variable Selector/1
  FT_PMGB/1 -> Terminator3/1

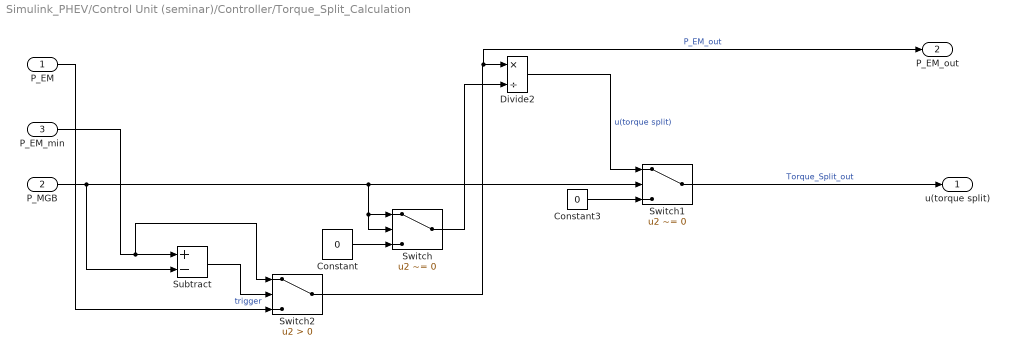
== system Simulink_PHEV/Control Unit (seminar)/Controller/Torque_Split_Calculation ==
  P_EM : Inport
  P_MGB : Inport  Port=2
  P_EM_min : Inport  Port=3
  Constant : Constant  Value=0
  Constant3 : Constant  Value=0
  Divide2 : Product  Inputs=*/
  Subtract : Sum  Inputs=+-
  Switch : Switch  Criteria=u2 ~= 0  SaturateOnIntegerOverflow=off  InputSameDT=off
  Switch1 : Switch  Criteria=u2 ~= 0  SaturateOnIntegerOverflow=off  InputSameDT=off
  Switch2 : Switch  Criteria=u2 > Threshold  SaturateOnIntegerOverflow=off  InputSameDT=off
  u(torque split) : Outport
  P_EM_out : Outport  Port=2
  wires:
  Constant/1 -> Switch/3
  Switch/1 -> Divide2/2
  Constant3/1 -> Switch1/3
  Divide2/1 -> Switch1/1  "u(torque split)"
  Switch1/1 -> u(torque split)/1  "Torque_Split_out"
  Subtract/1 -> Switch2/2  "trigger"
  P_EM/1 -> Switch2/3
  Switch2/1 -> P_EM_out/1, Divide2/1  "P_EM_out"
  P_MGB/1 -> Subtract/2, Switch/2, Switch/1, Switch1/2
  P_EM_min/1 -> Switch2/1, Subtract/1

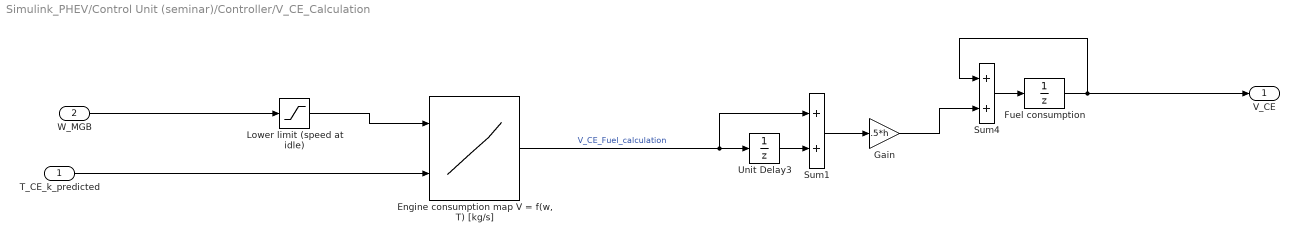
== system Simulink_PHEV/Control Unit (seminar)/Controller/V_CE_Calculation ==
  T_CE_k_predicted : Inport
  W_MGB : Inport  Port=2
  "Engine consumption map V = f(w, T) [kg/s]" : Lookup2D  RowIndex=w_CE_row  ColumnIndex=T_CE_col  Table=V_CE_map  SaturateOnIntegerOverflow=off  InputSameDT=off
  Fuel consumption : UnitDelay  SampleTime=h  HasFrameUpgradeWarning=on
  Gain : Gain  Gain=.5*h
  Lower limit (speed at idle) : Saturate  UpperLimit=inf  LowerLimit=105
  Sum1 : Sum  InputSameDT=on  SaturateOnIntegerOverflow=on  OutDataTypeStr=Inherit: Same as first input
  Sum4 : Sum  InputSameDT=on  SaturateOnIntegerOverflow=on  OutDataTypeStr=Inherit: Same as first input
  Unit Delay3 : UnitDelay  SampleTime=h  HasFrameUpgradeWarning=on
  V_CE : Outport
  wires:
  T_CE_k_predicted/1 -> "Engine consumption map V = f(w, T) [kg/s]"/2
  W_MGB/1 -> Lower limit (speed at idle)/1
  Sum4/1 -> Fuel consumption/1
  Sum1/1 -> Gain/1
  "Engine consumption map V = f(w, T) [kg/s]"/1 -> Sum1/1, Unit Delay3/1  "V_CE_Fuel_calculation"
  Gain/1 -> Sum4/2
  Unit Delay3/1 -> Sum1/2
  Lower limit (speed at idle)/1 -> "Engine consumption map V = f(w, T) [kg/s]"/1
  Fuel consumption/1 -> Sum4/1, V_CE/1

== matlab function Simulink_PHEV/Control Unit (seminar)/Controller/MATLAB Function2 ==
  data: PMGB input; y output
function y = fcn(PMGB)

if PMGB > 0
    ref_Q_BT = 3600;
else
    ref_Q_BT = 32000;
end
y = [ref_Q_BT 0.01];

== stateflow chart Simulink_PHEV/Control Unit (seminar)/Controller/Operation_Modes ==
  state Regeneration
    entry:
    OFF_States = 0;
    LPS = 0;
    ED=0;
    REG=1;
  state Load_Point_Shifting
    entry:
    OFF_States = 0;
    LPS = 1;
    ED=0;
    REG=0;
  state OFF
    entry:
    OFF_States = 1;
    LPS = 0;
    ED=0;
    REG=0;
    OFF -> OFF [order 1]
  state Electric_Driving
    entry:
    OFF_States = 0;
    LPS = 0;
    ED=1;
    REG=0;
  Load_Point_Shifting -> Regeneration [order 2] : [(T_MGB <0 & u == 1) | (T_MGB < 0 & 0 <= u & u < 1)]
  Regeneration -> Load_Point_Shifting [order 1] : [[(T_MGB >0 & 0 <= u & u < 1) | (T_MGB > 0 & u < 0)]]
  (default) -> OFF
  Load_Point_Shifting -> OFF [order 3] : [T_MGB == 0 & u == 0]
  Regeneration -> OFF [order 3] : [T_MGB == 0 & u == 0]
  OFF -> Load_Point_Shifting [order 1] : [[(T_MGB >0 & 0 <= u & u < 1) | (T_MGB > 0 & u < 0)]]
  OFF -> Regeneration [order 2] : [[(T_MGB <0 & u == 1) | (T_MGB < 0 & 0 <= u & u < 1)]]
  Electric_Driving -> OFF [order 3] : [T_MGB == 0 & u == 0]
  OFF -> Electric_Driving [order 3] : [[T_MGB > 0 & u == 1]]
  Electric_Driving -> Load_Point_Shifting [order 2] : [(T_MGB >0 & 0 <= u & u < 1) | (T_MGB > 0 & u < 0)]
  Load_Point_Shifting -> Electric_Driving [order 1] : [T_MGB > 0 & u== 1]
  Electric_Driving -> Regeneration [order 1] : [(T_MGB <0 & u == 1) | (T_MGB < 0 & 0 <= u & u < 1)]
  Regeneration -> Electric_Driving [order 2] : [T_MGB > 0 & u == 1]
  data: T_MGB input; u input; OFF_States local; LPS local; ED local; REG local

== matlab function Simulink_PHEV/Control Unit (seminar)/Controller/MATLAB Function ==
  data: T_MGB input; MV_seq input; P_EM_out input; T_CE_k_plus_1 output; w_MGB input; T_EM_k_plus_1 output
function [T_CE_k_plus_1,T_EM_k_plus_1] = fcn(T_MGB, MV_seq,P_EM_out, w_MGB)
T_EM_k_plus_1 = 0;
PCE_K_plus_1 = MV_seq(2,2);
PEM_K_plus_1 = MV_seq(2,1);
if w_MGB > 105
    T_CE_k_plus_1 = PCE_K_plus_1/w_MGB;
else
    T_CE_k_plus_1 = 0;
end
if T_MGB >=0
    if w_MGB == 0
        T_EM_k_plus_1 = 0;
    else 
        T_EM_k_plus_1 = PEM_K_plus_1/w_MGB;
    end
else
    if w_MGB ~= 0
        T_EM_k_plus_1 = P_EM_out/w_MGB;
    else
    end

end

end

== matlab function Simulink_PHEV/Control Unit (seminar)/Controller/Input_Constraints/MATLAB Function1 ==
  data: T_MGB input; dw_MGB input; T_max_CE input; w_MGB input; U_min output; T_max_EM input; U_max output; Q_BT input; debug_max output; debug_min output; eta_EM input
function [U_min,U_max,debug_max,debug_min] = Input_Constraints(T_MGB, dw_MGB, T_max_CE, w_MGB, T_max_EM, Q_BT, eta_EM)


delta_t = 1;
delta_p = delta_t * w_MGB;
theta_CE = 0.2;
theta_EM = 0.1;


% Battery Parameters
c_BT_E1     =  39;                          % Minimum battery voltage for discharging (13 cells, 3 V/cell, seminar)                 [V]
c_BT_E2     =  0.013;					    % Minimum battery resistance for discharging (13 cells, 1 mOhm/cell, seminar)           [Ohm]
c_BT_E3     =  15.6;					    % Maximum battery voltage variation for discharging (13 cells, 1.2 V/cell, seminar)     [V]
c_BT_E4     =  0;							% Minimum battery resistance variation for discharging (13 cells, 0 mOhm/cell, seminar) [Ohm]
c_BT_L1     =  c_BT_E1;                     % c_BT_L1 = c_BT_EL1 for continuity reasons
c_BT_L2     =  0.013;					    % Minimum battery resistance for charging (13 cells, 1 mOhm/cell, seminar)              [V]
c_BT_L3     =  c_BT_E3;                     % c_BT_L3 = c_BT_EL3 for continuity reasons
c_BT_L4     =  0.00;                        % Minimum battery resistance variation for charging (13 cells, 0 mOhm/cell, seminar)    [Ohm]

I_0 = 10;

Q_bt0      = I_0 * 3600;					% Discharge current in 1 h              [C]
I_bt_max    = (60/2)*I_0;			    	% Maximum charge/discharge current      [A]
%eta_EM = 1; 

%%
% During discharging 
AE1_discharge = (c_BT_E3 * (Q_BT/Q_bt0)) + c_BT_E1;
AE2_discharge = (c_BT_E4) * (Q_BT/Q_bt0) + c_BT_E2;
P_BT_discharge = I_bt_max^2 * ((AE1_discharge/I_bt_max) - (AE2_discharge/I_0));

% During charging
AE1_charge = (c_BT_L3 * (Q_BT/Q_bt0)) + c_BT_L1;
AE2_charge = (c_BT_L4) * (Q_BT/Q_bt0) + c_BT_L2;
P_BT_charge = -(I_bt_max^2 * ((AE1_charge/I_bt_max) - (AE2_charge/I_0)));




%% CE Constraints
T_CE_inertia = abs(theta_CE* dw_MGB);       % Inertial Torque of CE
% Upper Limit of P_CE
T_CE_upper = T_max_CE-delta_t -T_CE_inertia;
P_CE_max = T_CE_upper*w_MGB;

% Lower Limit of P_CE 
P_CE_min = 0;
  

%% EM Constraints

T_EM_inertia = abs(theta_EM* dw_MGB);
% Upper Limit of P_EM

    if w_MGB > 0
        T_EM_upper = T_max_EM - T_EM_inertia - delta_t;
    else
        T_EM_upper = T_max_EM -T_EM_inertia;                % delta is not include because at w_MGB =0, T_EM should be 0
    end
    
P_EM_lim_max = T_EM_upper * w_MGB;
P_em_cur_max = P_BT_discharge/eta_EM - (T_EM_inertia * w_MGB);
P_EM_max = min(P_EM_lim_max,P_em_cur_max-delta_p);


% Lower Limit of P_EM
if T_MGB >=0
    T_EM_lower = -T_EM_upper;
else
    T_EM_lower = max(T_MGB+delta_t, -T_EM_upper);
end

P_EM_lim_min = T_EM_lower * w_MGB;


P_em_cur_min = P_BT_charge/eta_EM -(T_EM_inertia*w_MGB);
P_EM_min = max(P_EM_lim_min,P_em_cur_min+delta_p);

debug_max = [P_EM_lim_max,P_BT_discharge,P_em_cur_max];
debug_min = [P_EM_lim_min,P_BT_charge,P_em_cur_min];
U_min = [P_EM_min;P_CE_min];
U_max = [P_EM_max;P_CE_max];
